simulink model "LinMotAct_total"  (R2019b)
settings: Solver=FixedStepAuto  StartTime=0.0  StopTime=inf  FixedStep=0.001  RelTol=1e-3  EnableMultiTasking=on
PostLoadFcn:
  | if any(exist('dsrtsu_mdlpostloadfcn', 'file') ~= 0), dsrtsu_mdlpostloadfcn('Execute', bdroot); end
values from neighbouring files (symbols this model uses):
  Ts_Outer = 0.1    [Working_model_LastVersion24_June.m]    (also in model_and_controller.m)
undefined symbols (not defined in the file or in its folder): denc_mi, denco13_dis_des, denF, numc_mi, numco13_dis_des, numF
libraries: rti3002t2lib x6, simulink x4, rtilibm x3, rti4201serlib x3
(part 1 of 2)
settings Model: DSRTSU_INTERNAL_RTI_VER=550  DSRTSU_INTERNAL_RTI_TYPE=rti1005  RTICANMMDATA=struct('GeneralSetupData',struct('modelroot','C:\Ball_and_Plate\Actuator_Control','generalsettings',struct('filesettings',struct('destfolder',struct('Name','RTICANMM_FILES','Check',1),'buildfolder',struct('Name','.','Check',1),'AbsDestfolder',struct('Name','C:\Ball_and_Plate\Actuator_Control\RTICANMM_FILES'),'AbsBuildfolder',struct('Name','C:\Ball_and_Plate\Actuator_Control'))),'options',struct('addpaths',1,'rmpaths',1,'addtrcexclusion',true,'cannavigator',struct('checkmonitoring',0),'show_usrtrc',0,'use_usrtrc',0),'advanced',struct('options',ones(1,100)),'MPSetup',{{}},'RTI',struct('Type','RTI1005','Ver','7.13','Date','02-Nov-2019'),'modelname','LinMotAct_total','block','LinMotAct_total'))  DSRTSU_INTERNAL_RTIFPGA=150  ExtModeArmWhenConnect=off  Creator=s060699  LastModifiedBy=20193994
settings SolverCC: AutoInsertRateTranBlk=on
settings DataIOCC: LimitDataPoints=on  SaveFormat=Array  SignalLoggingSaveFormat=ModelDataLogs  ReturnWorkspaceOutputs=off  SignalLoggingName=sigsOut
settings OptimizationCC: BlockReduction=off  ConditionallyExecuteInputs=off  OptimizeBlockIOStorage=off  BufferReuse=off  GlobalBufferReuse=off  ExpressionFolding=off  ExpressionDepthLimit=2147483647  LocalBlockOutputs=off  InitFltsAndDblsToZero=on  LifeSpan=inf  OptimizeDataStoreBuffers=off  BusAssignmentInplaceUpdate=off
settings DebuggingCC: SaveWithParameterizedLinksMsg=none  UnderspecifiedInitializationDetection=Classic  MergeDetectMultiDrivingBlocksExec=none  SignalResolutionControl=TryResolveAllWithWarning  MultiTaskDSMMsg=warning  MultiTaskCondExecSysMsg=none  FcnCallInpInsideContextMsg=warning  StateNameClashWarn=warning  SFUnexpectedBacktrackingDiag=warning  SFNoUnconditionalDefaultTransitionDiag=warning  SFExecutionAtInitializationDiag=none  ArithmeticOperatorsInVariantConditions=warning
settings HardwareCC: ProdBitPerPointer=32  ProdBitPerSizeT=32  ProdBitPerPtrDiffT=32  ProdLargestAtomicInteger=Integer  ProdEndianess=BigEndian  ProdWordSize=32  ProdHWDeviceType=Custom Processor->Custom  TargetIntDivRoundTo=Zero  TargetEndianess=BigEndian  TargetHWDeviceType=Custom Processor->Custom
settings ModelReferenceCC: PropagateSignalLabelsOutOfModel=off
settings SFSimCC: MATLABDynamicMemAlloc=off
settings RTWCC: Description=dSPACE DS1005 Hardware Platform  SystemTargetFile=rti1005.tlc  MakeCommand=make_rti  TemplateMakefile=rti1005.tmf  RTWVerbose=off  RetainRTWFile=on
settings CodeAppCC: CustomSymbolStrField=$H$N$M  CustomSymbolStrFcn=$R$H$N$M$F  StateflowObjectComments=on
settings STFCustomTargetCC: TargetFcnLib=ansi_tfl_tmw.mat  ParMdlRefBuildCompliant=on  CPPClassGenCompliant=on  SystemTargetFile=rti1005.tlc
settings GRTTargetCC: TargetFcnLib=ansi_tfl_tmw.mat  TargetLangStandard=C89/C90 (ANSI)  CompOptLevelCompliant=off  ConcurrentExecutionCompliant=off  CombineOutputUpdateFcns=off  MatFileLogging=off  UseToolchainInfoCompliant=off  ExtModeMexFile=rti_comm_2
settings ConfigComp: CovMetricSettings=dw  CovHtmlReporting=on  CovSaveCumulativeToWorkspaceVar=on  CovSaveSingleToWorkspaceVar=on

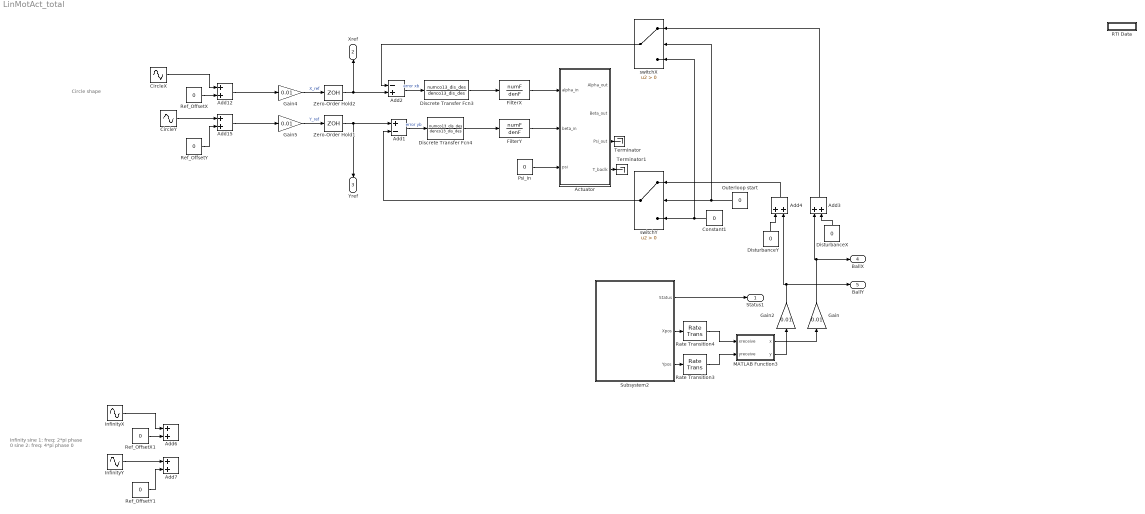
== system LinMotAct_total ==
  note: Infinity
      | sine 1: freq: 2*pi   phase 0
      | sine 2: freq: 4*pi   phase 0
  note: Circle shape
  Actuator : Subsystem
  Add1 : Sum  Inputs=+-
  Add{3..4,6..7,12,15} (6 alike) : Sum
  Add2 : Sum  Inputs=-+
  CircleX : Sin  Amplitude=0  Frequency=0.8  SampleTime=0
  CircleY : Sin  Amplitude=0  Frequency=0.8  Phase=pi/2  SampleTime=0
  Constant1 : Constant  Value=0
  Discrete Transfer Fcn3 : DiscreteTransferFcn  Numerator=numco13_dis_des  Denominator=denco13_dis_des
  Discrete Transfer Fcn4 : DiscreteTransferFcn  Numerator=numco13_dis_des  Denominator=denco13_dis_des
  DisturbanceX : Constant  Value=0
  DisturbanceY : Constant  Value=0
  FilterX : TransferFcn  Numerator=numF  Denominator=denF
  FilterY : TransferFcn  Numerator=numF  Denominator=denF
  Gain{,2,4..5} (4 alike) : Gain  Gain=0.01
  InfinityX : Sin  Amplitude=0  Frequency=1.41  SampleTime=0
  InfinityY : Sin  Amplitude=0  Frequency=2.82  SampleTime=0
  MATLAB Function3 : MATLAB Function  TreatAsAtomicUnit=on
  Outerloop start : Constant  Value=0
  Psi_in : Constant  Value=0
  RTI Data : Subsystem  Tag=struct('RTIDataServer',struct('RTIDataServerVs','2','RTIModelDescription','struct(''main'',''LinMotAct_total'',''sub'','''',''isMp'',0)'))  LoadFcn="if exist('rtidc'), try,  rtidc('DataHostBlockClbLoad', gcbh); catch, disp(['Warning: ''LoadFcn'' for RTI Data block failed: ' lasterr]); end, end,"  mask(RTI_DATA_HOST){}
      mask help:
      | RTI Data Block.
      | This block is used by RTI to store internal model-dependent data.
      | Please keep this block on the root level of the model. Deleting this block will result in data loss.
      |
      | NEVER DELETE OR COPY THIS BLOCK!
      settings: CopyFcn="if exist('rtidc'), try,  rtidc('DataHostBlockClbCopy', gcbh); catch, disp(['Warning: ''CopyFcn'' for RTI Data block failed: ' lasterr]); end, end,"  DeleteFcn="if exist('rtidc'), try,  rtidc('DataHostBlockClbDelete', gcbh); catch, disp(['Warning: ''DeleteFcn'' for RTI Data block failed: ' lasterr]); end, end,"  ModelCloseFcn="if exist('rtidc'), try,  rtidc('DataHostBlockClbModelClose', gcbh); catch, disp(['Warning: ''ModelCloseFcn'' for RTI Data block failed: ' lasterr]); end, end,"  PreSaveFcn="if exist('rtidc'), try,  rtidc('DataHostBlockClbPreSave', gcbh); catch, disp(['Warning: ''PreSaveFcn'' for RTI Data block failed: ' lasterr]); end, end,"  PostSaveFcn="if exist('rtidc'), try,  rtidc('DataHostBlockClbPostSave', gcbh); catch, disp(['Warning: ''PostSaveFcn'' for RTI Data block failed: ' lasterr]); end, end,"  NameChangeFcn="if exist('rtidc'), try,  rtidc('DataHostBlockClbNameChange', gcbh); catch, disp(['Warning: ''NameChangeFcn'' for RTI Data block failed: ' lasterr]); end, end,"
      mask Help:
      | RTI Data Block.
      | This block is used by RTI to store internal model-dependent data.
      | Please keep this block on the root level of the model. Deleting this block will result in data loss.
      | 
      | NEVER DELETE OR COPY THIS BLOCK!
      mask Display:
      | text(0.5, 0.5, 'RTI Data', 'HorizontalAlignment', 'center');
      | plot([1 0]);
  Rate Transition3 : RateTransition  Deterministic=off  OutPortSampleTimeMultiple=Ts_Outer  OutPortSampleTime=Ts_Outer
  Rate Transition4 : RateTransition  Deterministic=off  OutPortSampleTimeMultiple=Ts_Outer  OutPortSampleTime=Ts_Outer
  Ref_OffsetX : Constant  Value=0
  Ref_OffsetX1 : Constant  Value=0
  Ref_OffsetY : Constant  Value=0
  Ref_OffsetY1 : Constant  Value=0
  Subsystem2 : Subsystem
  Terminator : Terminator
  Terminator1 : Terminator
  Zero-Order Hold1 : ZeroOrderHold  SampleTime=Ts_Outer
  Zero-Order Hold2 : ZeroOrderHold  SampleTime=Ts_Outer
  switchX : Switch  Criteria=u2 > Threshold
  switchY : Switch  Criteria=u2 > Threshold
  Status1 : Outport
  Xref : Outport  Port=2
  Yref : Outport  Port=3
  BallX : Outport  Port=4
  BallY : Outport  Port=5
  wires:
  Ref_OffsetY/1 -> Add15/2
  CircleY/1 -> Add15/1
  Ref_OffsetX/1 -> Add12/2
  CircleX/1 -> Add12/1
  Gain4/1 -> Zero-Order Hold2/1  "X_ref"
  Gain5/1 -> Zero-Order Hold1/1  "Y_ref"
  Psi_in/1 -> Actuator/3(psi)
  Actuator/3(Psi_out) -> Terminator/1
  Actuator/4(T_baclk) -> Terminator1/1
  Subsystem2/1(Status) -> Status1/1
  Subsystem2/3(Ypos) -> Rate Transition3/1
  Subsystem2/2(Xpos) -> Rate Transition4/1
  Rate Transition3/1 -> MATLAB Function3/2(yreceive)
  Rate Transition4/1 -> MATLAB Function3/1(xreceive)
  MATLAB Function3/1(x) -> Gain/1
  Add2/1 -> Discrete Transfer Fcn3/1  "error xb"
  Add1/1 -> Discrete Transfer Fcn4/1  "error yb"
  Zero-Order Hold2/1 -> Add2/2, Xref/1
  Zero-Order Hold1/1 -> Add1/1, Yref/1
  Outerloop start/1 -> switchY/2, switchX/2
  Constant1/1 -> switchX/3, switchY/3
  Gain/1 -> Add3/1, BallX/1
  MATLAB Function3/2(y) -> Gain2/1
  DisturbanceX/1 -> Add3/2
  DisturbanceY/1 -> Add4/1
  switchY/1 -> Add1/2
  switchX/1 -> Add2/1
  Add4/1 -> switchY/1
  Add3/1 -> switchX/1
  Gain2/1 -> Add4/2, BallY/1
  FilterX/1 -> Actuator/1(alpha_in)
  FilterY/1 -> Actuator/2(beta_in)
  Ref_OffsetX1/1 -> Add6/2
  InfinityX/1 -> Add6/1
  Ref_OffsetY1/1 -> Add7/2
  InfinityY/1 -> Add7/1
  Add12/1 -> Gain4/1
  Add15/1 -> Gain5/1
  Discrete Transfer Fcn3/1 -> FilterX/1
  Discrete Transfer Fcn4/1 -> FilterY/1

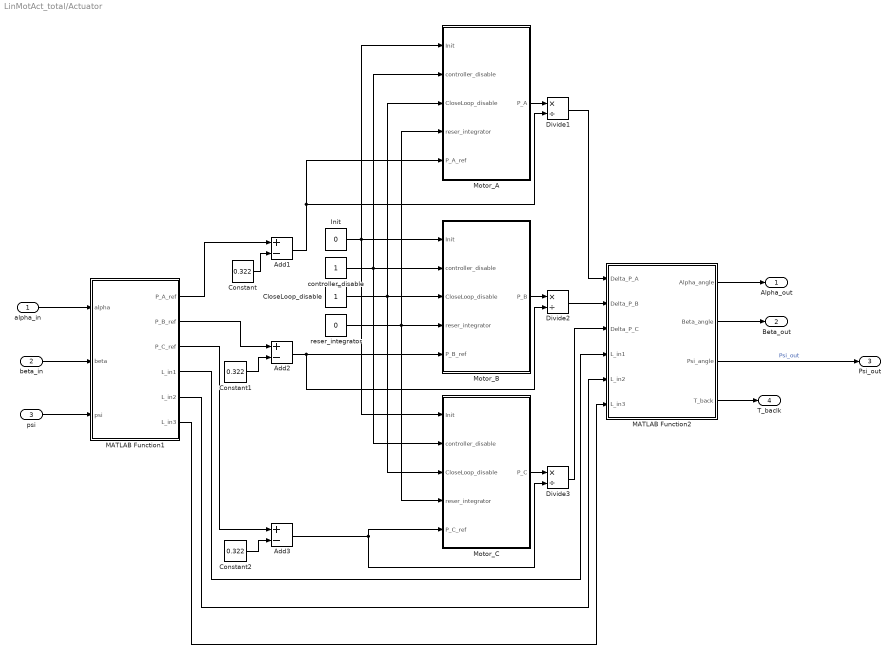
== system LinMotAct_total/Actuator ==
  alpha_in : Inport
  beta_in : Inport  Port=2
  psi : Inport  Port=3
  Add1 : Sum  Inputs=+-
  Add2 : Sum  Inputs=+-
  Add3 : Sum  Inputs=+-
  CloseLoop_disable : Constant
  Constant : Constant  Value=0.322
  Constant1 : Constant  Value=0.322
  Constant2 : Constant  Value=0.322
  Divide1 : Product  Inputs=*/
  Divide2 : Product  Inputs=*/
  Divide3 : Product  Inputs=*/
  "Init " : Constant  Value=0
  MATLAB Function1 : MATLAB Function  TreatAsAtomicUnit=on
  MATLAB Function2 : MATLAB Function  TreatAsAtomicUnit=on
  Motor_A : Subsystem
  Motor_B : Subsystem
  Motor_C : Subsystem
  controller_disable : Constant
  reser_integrator : Constant  Value=0
  Alpha_out : Outport
  Beta_out : Outport  Port=2
  Psi_out : Outport  Port=3
  T_baclk : Outport  Port=4
  wires:
  Motor_B/1(P_B) -> Divide2/1
  "Init "/1 -> Motor_C/1(Init), Motor_A/1(Init), Motor_B/1(Init)
  Divide3/1 -> MATLAB Function2/3(Delta_P_C)
  controller_disable/1 -> Motor_A/2(controller_disable), Motor_B/2(controller_disable), Motor_C/2(controller_disable)
  Add3/1 -> Motor_C/5(P_C_ref), Divide3/2
  MATLAB Function1/1(P_A_ref) -> Add1/1
  reser_integrator/1 -> Motor_A/4(reser_integrator), Motor_C/4(reser_integrator), Motor_B/4(reser_integrator)
  MATLAB Function1/3(P_C_ref) -> Add3/1
  MATLAB Function1/5(L_in2) -> MATLAB Function2/5(L_in2)
  Divide1/1 -> MATLAB Function2/1(Delta_P_A)
  Motor_C/1(P_C) -> Divide3/1
  MATLAB Function2/1(Alpha_angle) -> Alpha_out/1
  psi/1 -> MATLAB Function1/3(psi)
  Add2/1 -> Divide2/2, Motor_B/5(P_B_ref)
  Motor_A/1(P_A) -> Divide1/1
  MATLAB Function2/4(T_back) -> T_baclk/1
  Add1/1 -> Motor_A/5(P_A_ref), Divide1/2
  Constant1/1 -> Add2/2
  beta_in/1 -> MATLAB Function1/2(beta)
  Constant/1 -> Add1/2
  Constant2/1 -> Add3/2
  Divide2/1 -> MATLAB Function2/2(Delta_P_B)
  MATLAB Function1/6(L_in3) -> MATLAB Function2/6(L_in3)
  CloseLoop_disable/1 -> Motor_A/3(CloseLoop_disable), Motor_C/3(CloseLoop_disable), Motor_B/3(CloseLoop_disable)
  MATLAB Function1/2(P_B_ref) -> Add2/1
  MATLAB Function1/4(L_in1) -> MATLAB Function2/4(L_in1)
  MATLAB Function2/2(Beta_angle) -> Beta_out/1
  MATLAB Function2/3(Psi_angle) -> Psi_out/1  "Psi_out"
  alpha_in/1 -> MATLAB Function1/1(alpha)

== system LinMotAct_total/RTI Data ==
  RTI Data Store : Subsystem  Tag="struct('private',struct('version',struct('dsVer',uint32(2),'dsVerCreation',uint32(2),'RTI',struct('ver','7.13','type','RTI1005')),'access',struct('type','Model','isPerm',1,'created',['07-Jul-2020 15:56:35'],'modified',['31-Jul-2020 14:12:37'],'location','')),'public',struct('main',struct('data',[]),'sub',struct('name',{{'LinMotAct_total'}},'data',{{struct('TH',struct('thTaskInfo',struct('taskType',{'TIMER','HWINT','TMRINT','SWINT','GLINT'},'tasksNumOf',{2,0,0,0,0},'srcIds',{{'TIMERA','TIMERA2'},{},{},{},{}},'taskNames',{{['Timer Task 1'],['Timer Task 2']},{},{},{},{}})),'th_tc',struct('dataType',{'TASK','TASK'},'taskGroupId',{'',''},'taskGroupList',{{},{}},'taskSchedulingPolicy',{'FCFS','FCFS'},'taskType',{'TIMER','TIMER'},'blkh',{-1,-1},'srcId',{'TIMERA','TIMERA2'},'srcSgnName',{['Timer A interrupt'],['Timer Task 1']},'srcCpuName',{'',''},'taskName',{['Timer Task 1  [0.001] s'],['Timer Task 2  [0.1] s']},'taskNameDisplayExt',{'',''},'smplTime',{0.001,0.1},'smplTimeOffs',{0,0},'hasFixedPriority',{0,0},'priority',{1,2},'hasFixedOvc',{0,0},'ovcType',{1,1},'ovcMax',{1,1}),'tc_th',struct('dataType',{'TASK','TASK'},'taskGroupId',{'',''},'taskGroupList',{{},{}},'taskSchedulingPolicy',{'FCFS','FCFS'},'taskType',{'TIMER','TIMER'},'blkh',{-1,-1},'srcId',{'TIMERA','TIMERA2'},'srcSgnName',{['Timer A interrupt'],['Timer Task 1']},'srcCpuName',{'',''},'taskName',{['Timer Task 1  [0.001] s'],['Timer Task 2  [0.1] s']},'taskNameDisplayExt',{'',''},'smplTime',{0.001,0.1},'smplTimeOffs',{0,0},'hasFixedPriority',{0,0},'priority',{1,2},'hasFixedOvc',{0,0},'ovcType',{1,1},'ovcMax',{1,1}))}})))"  mask(RTI_DATA_STORE){}
      mask help:
      | RTI Data Store Block. This block is used by RTI to store internal model dependent data. Deleting this block will result in data loss.
      |
      | NEVER DELETE, COPY, OR MODIFY THIS BLOCK!
      mask Help:
      | RTI Data Store Block. This block is used by RTI to store internal model dependent data. Deleting this block will result in data loss.
      | 
      | NEVER DELETE, COPY, OR MODIFY THIS BLOCK!
      mask Display: text(0.5, 0.5, ' ', 'HorizontalAlignment', 'center');

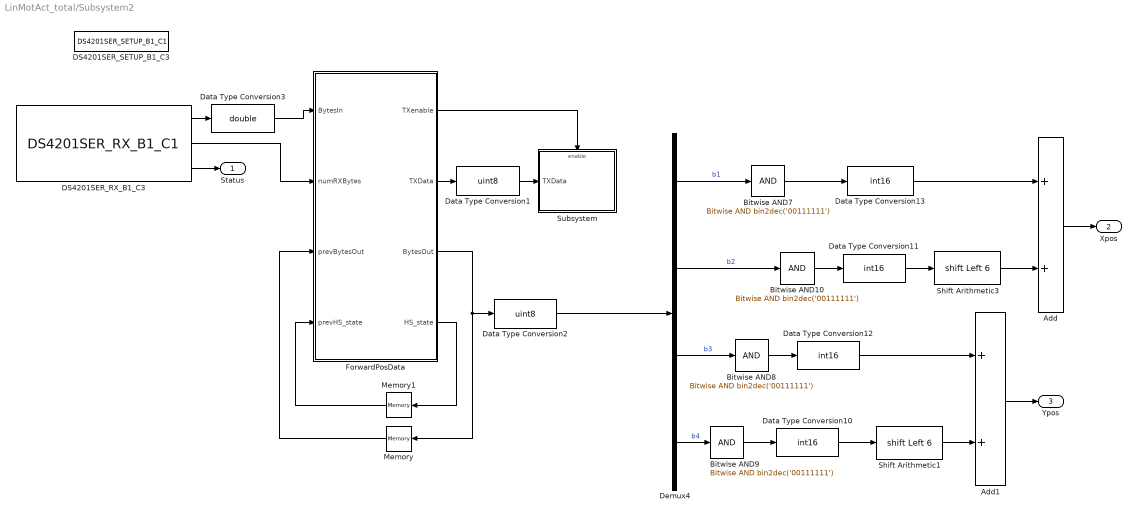
== system LinMotAct_total/Subsystem2 ==
  Add : Sum
  Add1 : Sum
  Bitwise AND{7..10} (4 alike) : simulink/Logic and Bit Operations/Bitwise Operator  logicop=AND  UseBitMask=on  BitMask=bin2dec('00111111')  BitMaskRealWorld=Stored Integer
  DS4201SER_RX_B1_C3 : rti4201serlib/DS4201SER_RX_B1_C1  Reserved1=[]  Reserved2=[]  Reserved3=[]  Reserved4=[]  DSProperties=struct('RTI',struct('IOBoardType',{{'DS4201','SER'}},'SlaveProcessor','NONE','Version',uint32(1),'BlockType',struct('isSLSource',uint8(1),'isSLSink',uint8(1),'isHWSource',uint8(0),'isHWSink',uint8(1),'isSetup',uint8(0),'isInline',uint8(1),'isNonInline',uint8(0),'isInterrupt',uint8(0),'isChannelwise',uint8(1)),'UnitType','GENSER','Identifier','RECEIVE','DialogType','ML','BlockSet','NONE'))  RTIBlockInterface=struct('BlockName',struct('Token',{{'DS4201SER_RX_B','_C'}},'BlockParam',{{'BoardNo','ChannelNo'}}),'InputPortsWidth',int32(1),'InputPortsActive',0,'InputPortsDataType',{{'SS_UINT32'}},'InputPortsName',{{'NumBytes'}},'OutputPortsWidth',int32([4 1 1]),'OutputPortsActive',[1 1 1],'OutputPortsDataType',{{'SS_UINT8','SS_UINT32','SS_INT32'}},'OutputPortsName',{{'RXBytes','NumRXBytes','Status'}},'BlockDisplay',{{['Serial Receive'],'center'}},'IconTransparency','on','ParameterTunableNames',{{'BytesRefNumOf'}},'InitLevel',2,'DialogFcn','guigenserreceive','MaskDescription',['To read data from the UART SW FIFO.'])  RTIBlockParameters=struct('BoardNo',{{1,'ON',[1 16]}},'ChannelNo',{{3,'ON',[1 4]}},'ChannelNumOf',{{4,'OFF',[]}},'ReceptionDataMode',{{2,'OFF',[]}},'ParamTunableMode',{{1,'OFF',[]}},'BytesRefNumOfT',{{'4','OFF',[1 inf]}},'BytesRefNumOfNT',{{'4','OFF',[1 inf]}},'BytesRefNumOfMax',{{'4','OFF',[1 inf]}},'BytesRefNumOfMode',{{1,'OFF',[]}},'BytesActNumOfMode',{{1,'OFF',[]}},'ReceptionStatusMode',{{1,'OFF',[]}},'FifoSizeDefault',{{64,'OFF',[]}},'TLCFileName',{{'rtigenserreceive','OFF',[]}})  RTISFcnParameters=struct('BoardNo','double','ChannelNo','double','ChannelNumOf','double','ReceptionDataMode','double','ParamTunableMode','double','BytesRefNumOfT','double','BytesRefNumOfNT','double','BytesRefNumOfMax','double','BytesRefNumOfMode','double','BytesActNumOfMode','double','ReceptionStatusMode','double','TLCFileName','char')  RTIBlockParaDefault=struct('BoardNo',1,'ChannelNo',1,'ChannelNumOf',4,'ReceptionDataMode',1,'ParamTunableMode',1,'BytesRefNumOfT',1,'BytesRefNumOfNT',1,'BytesRefNumOfMax',1,'BytesRefNumOfMode',0,'BytesActNumOfMode',1,'ReceptionStatusMode',1,'FifoSizeDefault',64,'TLCFileName','rtigenserreceive')
  DS4201SER_SETUP_B1_C3 : rti4201serlib/DS4201SER_SETUP_B1_C1  Reserved1=[]  Reserved2=[]  Reserved3=[]  Reserved4=[]  DSProperties=struct('RTI',struct('Version',uint32(2),'IOBoardType',{{'DS4201','SER'}},'SlaveProcessor','NONE','BlockType',struct('isSLSource',uint8(0),'isSLSink',uint8(0),'isHWSource',uint8(0),'isHWSink',uint8(0),'isSetup',uint8(1),'isInline',uint8(1),'isNonInline',uint8(0),'isInterrupt',uint8(0),'isChannelwise',uint8(1)),'UnitType','GENSER','Identifier','SETUP','DialogType','ML','BlockSet','NONE'))  RTIBlockInterface=struct('BlockName',struct('Token',{{'DS4201SER_SETUP_B','_C'}},'BlockParam',{{'BoardNo','ChannelNo'}}),'BlockDisplay',{{['Serial Setup'],'center'}},'IconTransparency','off','ParameterTunableNames',{{}},'InitLevel',1,'DialogFcn','guigensersetup','MaskDescription',['To set the global specifications for the UART interface.'])  RTIBlockParameters=struct('ParityMode',{{1,'OFF',[1 3]}},'TransceiverMode',{{[3;1;3;1],'OFF',[]}},'QuartzFrequency',{{'24000000','OFF',[]}},'BoardNo',{{1,'ON',[1 16]}},'ChannelNo',{{3,'ON',[1 4]}},'ChannelNumOf',{{4,'OFF',[]}},'BaudRate',{{'9600','OFF',[]}},'DataBitsNumOf',{{4,'OFF',[1 4]}},'StopBitsNumOf',{{1,'OFF',[1 3]}},'ReceiveIntLevelUart',{{2,'OFF',[1 4]}},'AutoflowMode',{{0,'OFF',[]}},'FifoSize',{{'64','OFF',[]}},'ReceiveIntLevelFifo',{{0,'OFF',[]}},'FifoOverrunMode',{{2,'OFF',[]}},'FifoBlockSize',{{'4','OFF',[]}},'TermMode',{{0,'OFF',[]}},'TLCFileName',{{'rtigensersetup','OFF',[]}})  RTISFcnParameters=struct('BoardNo','double','ChannelNo','double','ChannelNumOf','double','BaudRate','double','DataBitsNumOf','double','StopBitsNumOf','double','ParityMode','double','TransceiverMode','double','ReceiveIntLevelUart','double','AutoflowMode','double','FifoSize','double','ReceiveIntLevelFifo','double','FifoBlockSize','double','TermMode','double','QuartzFrequency','double','TLCFileName','char')  RTIBlockParaDefault=struct('ParityMode',1,'TransceiverMode',[1;1;1;1],'QuartzFrequency',1843200,'BoardNo',1,'ChannelNo',1,'ChannelNumOf',4,'BaudRate',115200,'DataBitsNumOf',4,'StopBitsNumOf',1,'ReceiveIntLevelUart',4,'AutoflowMode',0,'FifoSize',64,'ReceiveIntLevelFifo',0,'FifoOverrunMode',1,'FifoBlockSize',0,'TermMode',1,'TLCFileName','rtigensersetup')
  Data Type Conversion1 : DataTypeConversion  OutDataTypeStr=uint8
  Data Type Conversion{10..13} (4 alike) : DataTypeConversion  OutDataTypeStr=int16
  Data Type Conversion2 : DataTypeConversion  OutDataTypeStr=uint8
  Data Type Conversion3 : DataTypeConversion  OutDataTypeStr=double
  Demux4 : Demux
  ForwardPosData : MATLAB Function  TreatAsAtomicUnit=on
  Memory : Memory  InitialCondition=[0 0 0 0]
  Memory1 : Memory
  Shift Arithmetic1 : ArithShift  BitShiftNumber=6  BitShiftDirection=Left
  Shift Arithmetic3 : ArithShift  BitShiftNumber=6  BitShiftDirection=Left
  Subsystem : Subsystem
  Status : Outport
  Xpos : Outport  Port=2
  Ypos : Outport  Port=3
  wires:
  Bitwise AND8/1 -> Data Type Conversion12/1
  Bitwise AND7/1 -> Data Type Conversion13/1
  Add/1 -> Xpos/1
  Add1/1 -> Ypos/1
  Bitwise AND10/1 -> Data Type Conversion11/1
  Bitwise AND9/1 -> Data Type Conversion10/1
  Data Type Conversion11/1 -> Shift Arithmetic3/1
  Data Type Conversion10/1 -> Shift Arithmetic1/1
  Data Type Conversion13/1 -> Add/1
  Data Type Conversion12/1 -> Add1/1
  Shift Arithmetic3/1 -> Add/2
  Shift Arithmetic1/1 -> Add1/2
  DS4201SER_RX_B1_C3/2 -> ForwardPosData/2(numRXBytes)
  DS4201SER_RX_B1_C3/3 -> Status/1
  ForwardPosData/3(BytesOut) -> Data Type Conversion2/1, Memory/1
  Memory/1 -> ForwardPosData/3(prevBytesOut)
  DS4201SER_RX_B1_C3/1 -> Data Type Conversion3/1
  ForwardPosData/4(HS_state) -> Memory1/1
  Memory1/1 -> ForwardPosData/4(prevHS_state)
  ForwardPosData/2(TXData) -> Data Type Conversion1/1
  ForwardPosData/1(TXenable) -> Subsystem/Enable
  Demux4/1 -> Bitwise AND7/1  "b1"
  Demux4/2 -> Bitwise AND10/1  "b2"
  Demux4/3 -> Bitwise AND8/1  "b3"
  Demux4/4 -> Bitwise AND9/1  "b4"
  Data Type Conversion1/1 -> Subsystem/1(TXData)
  Data Type Conversion2/1 -> Demux4/1
  Data Type Conversion3/1 -> ForwardPosData/1(BytesIn)

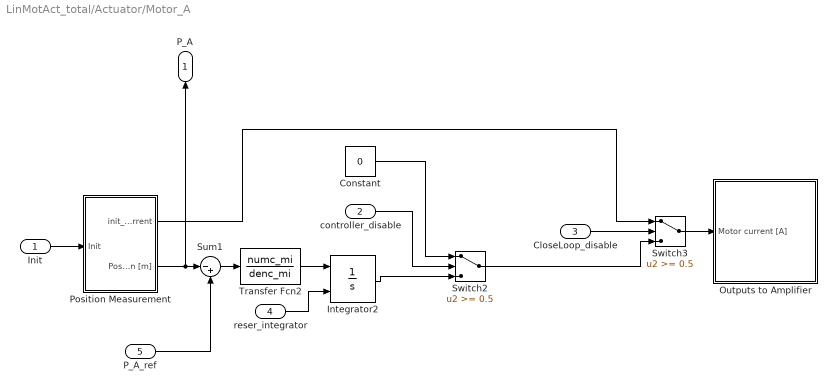
== system LinMotAct_total/Actuator/Motor_A ==
  Init : Inport
  controller_disable : Inport  Port=2
  CloseLoop_disable : Inport  Port=3
  reser_integrator : Inport  Port=4
  P_A_ref : Inport  Port=5
  Constant : Constant  Value=0
  Integrator2 : Integrator  ExternalReset=rising  LimitOutput=on  UpperSaturationLimit=2.7  LowerSaturationLimit=-2.7
  Outputs to Amplifier : Subsystem  TreatAsAtomicUnit=on
  Position Measurement : Subsystem  TreatAsAtomicUnit=on
  Sum1 : Sum  Inputs=|-+  SaturateOnIntegerOverflow=on
  Switch2 : Switch  Threshold=0.5
  Switch3 : Switch  Threshold=0.5
  Transfer Fcn2 : TransferFcn  Numerator=numc_mi  Denominator=denc_mi
  P_A : Outport
  wires:
  Integrator2/1 -> Switch2/3
  Switch3/1 -> Outputs to Amplifier/1(Motor current [A])
  Position Measurement/2(Position [m]) -> P_A/1, Sum1/1
  Position Measurement/1(init_current) -> Switch3/1
  Switch2/1 -> Switch3/3
  CloseLoop_disable/1 -> Switch3/2
  reser_integrator/1 -> Integrator2/2
  Sum1/1 -> Transfer Fcn2/1
  Constant/1 -> Switch2/1
  Transfer Fcn2/1 -> Integrator2/1
  controller_disable/1 -> Switch2/2
  P_A_ref/1 -> Sum1/2
  Init/1 -> Position Measurement/1(Init)

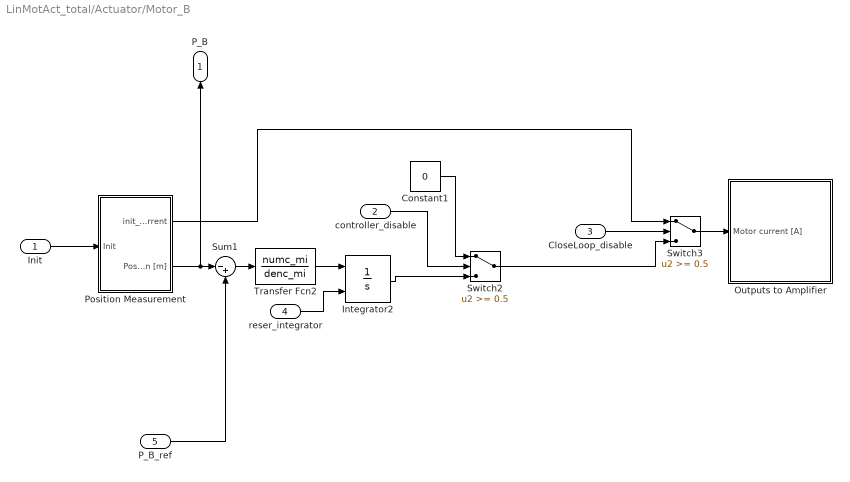
== system LinMotAct_total/Actuator/Motor_B ==
  Init : Inport
  controller_disable : Inport  Port=2
  CloseLoop_disable : Inport  Port=3
  reser_integrator : Inport  Port=4
  P_B_ref : Inport  Port=5
  Constant1 : Constant  Value=0
  Integrator2 : Integrator  ExternalReset=rising  LimitOutput=on  UpperSaturationLimit=2.7  LowerSaturationLimit=-2.7
  Outputs to Amplifier : Subsystem  TreatAsAtomicUnit=on
  Position Measurement : Subsystem  TreatAsAtomicUnit=on
  Sum1 : Sum  Inputs=|-+  SaturateOnIntegerOverflow=on
  Switch2 : Switch  Threshold=0.5
  Switch3 : Switch  Threshold=0.5
  Transfer Fcn2 : TransferFcn  Numerator=numc_mi  Denominator=denc_mi
  P_B : Outport
  wires:
  Integrator2/1 -> Switch2/3
  Switch3/1 -> Outputs to Amplifier/1(Motor current [A])
  Position Measurement/2(Position [m]) -> P_B/1, Sum1/1
  Position Measurement/1(init_current) -> Switch3/1
  Switch2/1 -> Switch3/3
  CloseLoop_disable/1 -> Switch3/2
  reser_integrator/1 -> Integrator2/2
  Sum1/1 -> Transfer Fcn2/1
  Transfer Fcn2/1 -> Integrator2/1
  controller_disable/1 -> Switch2/2
  P_B_ref/1 -> Sum1/2
  Constant1/1 -> Switch2/1
  Init/1 -> Position Measurement/1(Init)

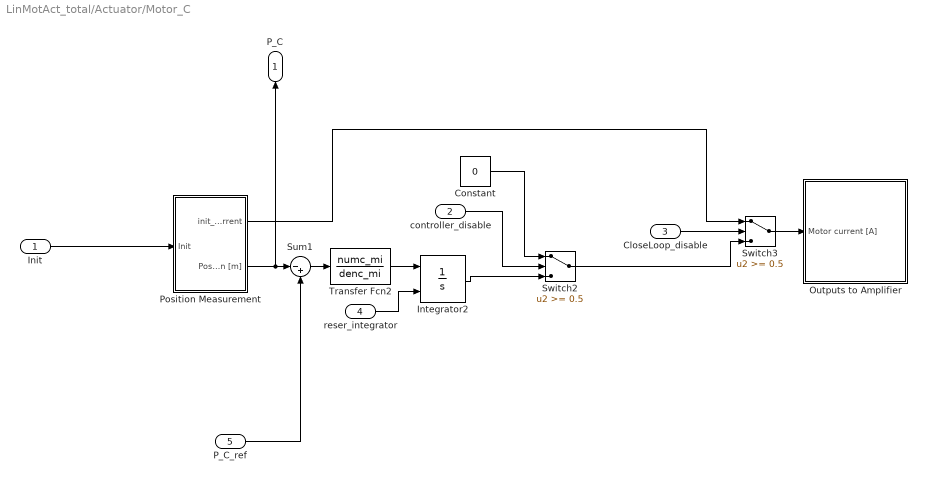
== system LinMotAct_total/Actuator/Motor_C ==
  Init : Inport
  controller_disable : Inport  Port=2
  CloseLoop_disable : Inport  Port=3
  reser_integrator : Inport  Port=4
  P_C_ref : Inport  Port=5
  Constant : Constant  Value=0
  Integrator2 : Integrator  ExternalReset=rising  LimitOutput=on  UpperSaturationLimit=2.7  LowerSaturationLimit=-2.7
  Outputs to Amplifier : Subsystem  TreatAsAtomicUnit=on
  Position Measurement : Subsystem  TreatAsAtomicUnit=on
  Sum1 : Sum  Inputs=|-+  SaturateOnIntegerOverflow=on
  Switch2 : Switch  Threshold=0.5
  Switch3 : Switch  Threshold=0.5
  Transfer Fcn2 : TransferFcn  Numerator=numc_mi  Denominator=denc_mi
  P_C : Outport
  wires:
  Integrator2/1 -> Switch2/3
  Switch3/1 -> Outputs to Amplifier/1(Motor current [A])
  Position Measurement/2(Position [m]) -> P_C/1, Sum1/1
  Position Measurement/1(init_current) -> Switch3/1
  Switch2/1 -> Switch3/3
  CloseLoop_disable/1 -> Switch3/2
  reser_integrator/1 -> Integrator2/2
  Sum1/1 -> Transfer Fcn2/1
  Constant/1 -> Switch2/1
  Transfer Fcn2/1 -> Integrator2/1
  controller_disable/1 -> Switch2/2
  P_C_ref/1 -> Sum1/2
  Init/1 -> Position Measurement/1(Init)

== system LinMotAct_total/RTI Data/RTI Data Store ==
  RTI Data Store : Subsystem  mask(RTI_DATA_STORE){}
      mask help:
      | RTI Data Store Block. This block is used by RTI to store internal model dependent data. Deleting this block will result in data loss.
      |
      | NEVER DELETE, COPY, OR MODIFY THIS BLOCK!
      mask Help:
      | RTI Data Store Block. This block is used by RTI to store internal model dependent data. Deleting this block will result in data loss.
      | 
      | NEVER DELETE, COPY, OR MODIFY THIS BLOCK!
      mask Display: text(0.5, 0.5, ' ', 'HorizontalAlignment', 'center');

== system LinMotAct_total/Subsystem2/Subsystem ==
  TXData : Inport
  Enable : EnablePort
  DS4201SER_TX_B1_C3 : rti4201serlib/DS4201SER_TX_B1_C1  Reserved1=[]  Reserved2=[]  Reserved3=[]  Reserved4=[]  DSProperties=struct('RTI',struct('IOBoardType',{{'DS4201','SER'}},'SlaveProcessor','NONE','Version',uint32(1),'BlockType',struct('isSLSource',uint8(1),'isSLSink',uint8(1),'isHWSource',uint8(1),'isHWSink',uint8(0),'isSetup',uint8(0),'isInline',uint8(1),'isNonInline',uint8(0),'isInterrupt',uint8(0),'isChannelwise',uint8(1)),'UnitType','GENSER','Identifier','TRANSMIT','DialogType','ML','BlockSet','NONE'))  RTIBlockInterface=struct('BlockName',struct('Token',{{'DS4201SER_TX_B','_C'}},'BlockParam',{{'BoardNo','ChannelNo'}}),'InputPortsWidth',int32([1 1]),'InputPortsActive',[1 0],'InputPortsDataType',{{'SS_UINT8','SS_UINT32'}},'InputPortsName',{{'TXBytes','NumBytes'}},'OutputPortsWidth',int32([1 1]),'OutputPortsActive',[1 1],'OutputPortsDataType',{{'SS_UINT32','SS_INT32'}},'OutputPortsName',{{'NumTXBytes','Status'}},'BlockDisplay',{{['Serial Transmit'],'center'}},'IconTransparency','on','ParameterTunableNames',{{'BytesRefNumOf'}},'InitLevel',2,'DialogFcn','guigensertransmit','MaskDescription',['To write data to the UART SW FIFO.'])  RTIBlockParameters=struct('BoardNo',{{1,'ON',[1 16]}},'ChannelNo',{{3,'ON',[1 4]}},'ChannelNumOf',{{4,'OFF',[]}},'TransmitFifoOverrunMode',{{1,'OFF',[]}},'ParamTunableMode',{{1,'OFF',[]}},'BytesRefNumOfT',{{'1','OFF',[1 inf]}},'BytesRefNumOfNT',{{'1','OFF',[1 inf]}},'BytesRefNumOfMax',{{'1','OFF',[1 inf]}},'BytesRefNumOfMode',{{1,'OFF',[]}},'BytesActNumOfMode',{{1,'OFF',[]}},'TransmissionStatusMode',{{1,'OFF',[]}},'FifoSizeDefault',{{64,'OFF',[]}},'TLCFileName',{{'rtigensertransmit','OFF',[]}})  RTISFcnParameters=struct('BoardNo','double','ChannelNo','double','ChannelNumOf','double','TransmitFifoOverrunMode','double','ParamTunableMode','double','BytesRefNumOfT','double','BytesRefNumOfNT','double','BytesRefNumOfMax','double','BytesRefNumOfMode','double','BytesActNumOfMode','double','TransmissionStatusMode','double','TLCFileName','char')  RTIBlockParaDefault=struct('BoardNo',1,'ChannelNo',1,'ChannelNumOf',4,'TransmitFifoOverrunMode',1,'ParamTunableMode',1,'BytesRefNumOfT',1,'BytesRefNumOfNT',1,'BytesRefNumOfMax',1,'BytesRefNumOfMode',0,'BytesActNumOfMode',1,'TransmissionStatusMode',1,'FifoSizeDefault',64,'TLCFileName','rtigensertransmit')
  Terminator : Terminator
  Terminator1 : Terminator
  wires:
  DS4201SER_TX_B1_C3/2 -> Terminator1/1
  DS4201SER_TX_B1_C3/1 -> Terminator/1
  TXData/1 -> DS4201SER_TX_B1_C3/1

== system LinMotAct_total/Actuator/Motor_A/Outputs to Amplifier ==
  Motor current [A] : Inport
  Current2V : Gain  Gain=10/3  SaturateOnIntegerOverflow=on  OutDataTypeStr=Inherit: Same as input  ParamDataTypeStr=Inherit: Same as input
  DS2102_B1 : rtilibm/DS2102/DS2102_B1  BoardNo=1  Range=[10 10 10 10 10 10]  IOErrorMode=[1 1 1 1 1 1]  DeglitcherMode=[0 0 0 0 0 0]  InitValue=[0 0 0 0 0 0]  TermMode=[1 1 1 1 1 1]  TermValue=[0 0 0 0 0 0]  DialogFcn=gui2102  UnitName={'DS2102_B'}  UnitValues={ 1 }  DSProperties=struct('RTI',struct('Version',uint32(1),'BlockType',struct('isSLSource',uint8(0),'isSLSink',uint8(1),'isHWSource',uint8(0),'isHWSink',uint8(1),'isSetup',uint8(0),'isInline',uint8(1),'isNonInline',uint8(0),'isInterrupt',uint8(0),'isChannelwise',uint8(0)),'IOBoardType','DS2102','UnitType','DAC','Identifier','DAC','DialogType','ML','BlockSet','NONE','SlaveProcessor','NONE'))
      settings: SourceProductName=dSPACE RTI1005
  DSPscale : Gain  Gain=1/10  SaturateOnIntegerOverflow=on  OutDataTypeStr=Inherit: Same as input  ParamDataTypeStr=Inherit: Same as input
  Saturation : Saturate  UpperLimit=3  LowerLimit=-3
  wires:
  Saturation/1 -> Current2V/1
  Current2V/1 -> DSPscale/1
  Motor current [A]/1 -> Saturation/1
  DSPscale/1 -> DS2102_B1/1

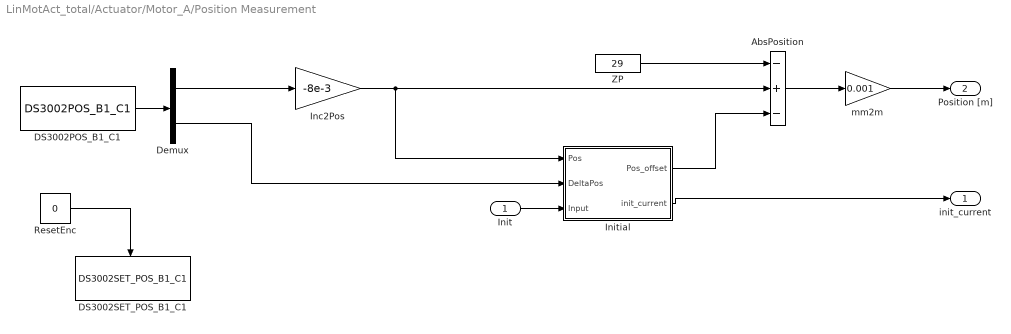
== system LinMotAct_total/Actuator/Motor_A/Position Measurement ==
  Init : Inport
  AbsPosition : Sum  Inputs=-+-  SaturateOnIntegerOverflow=on
  "DS3002POS_B1_C1 " : rti3002t2lib/DS3002POS_B1_C1  BoardNo=1  ChannelNo=1  LineSubdivNumOf=1  Reserved1=[]  Reserved2=[]  Reserved3=[]  Reserved4=[]  DialogFcn=gui3002pos_c_t2  UnitName={'DS3002POS_B', '_C'}  UnitValues="{ 1  1 }"  DSProperties=struct('RTI',struct('Version',uint32(1),'BlockType',struct('isSLSource',uint8(1),'isSLSink',uint8(0),'isHWSource',uint8(1),'isHWSink',uint8(0),'isSetup',uint8(0),'isInline',uint8(1),'isNonInline',uint8(0),'isInterrupt',uint8(0),'isChannelwise',uint8(1)),'IOBoardType','DS3002','UnitType','ENC','Identifier','ENCPOSCHT2','DialogType','ML','BlockSet','NONE','SlaveProcessor','NONE'))
  "DS3002SET_POS_B1_C1 " : rti3002t2lib/DS3002SET_POS_B1_C1  BoardNo=1  ChannelNo=1  PositionSetValue=0  Reserved1=[]  Reserved2=[]  Reserved3=[]  Reserved4=[]  DialogFcn=gui3002set_pos_c_t2  UnitName={'DS3002SET_POS_B', '_C'}  UnitValues="{ 1  1 }"  DSProperties=struct('RTI',struct('Version',uint32(1),'BlockType',struct('isSLSource',uint8(0),'isSLSink',uint8(1),'isHWSource',uint8(0),'isHWSink',uint8(0),'isSetup',uint8(0),'isInline',uint8(1),'isNonInline',uint8(0),'isInterrupt',uint8(0),'isChannelwise',uint8(1)),'IOBoardType','DS3002','UnitType','ENC','Identifier','ENCSETPOST2','DialogType','ML','BlockSet','NONE','SlaveProcessor','NONE'))
  Demux : Demux  Outputs=2
  Inc2Pos : Gain  Gain=-8e-3  SaturateOnIntegerOverflow=on  OutDataTypeStr=Inherit: Same as input  ParamDataTypeStr=Inherit: Same as input
  Initial : Subsystem
  ResetEnc : Constant  Value=0
  ZP : Constant  Value=29
  mm2m : Gain  Gain=0.001
  init_current : Outport  VectorParamsAs1DForOutWhenUnconnected=off
  Position [m] : Outport  Port=2  VectorParamsAs1DForOutWhenUnconnected=off
  wires:
  Demux/1 -> Inc2Pos/1
  AbsPosition/1 -> mm2m/1
  Inc2Pos/1 -> Initial/1(Pos), AbsPosition/2
  Initial/2(init_current) -> init_current/1
  mm2m/1 -> Position [m]/1
  Demux/2 -> Initial/2(DeltaPos)
  "DS3002POS_B1_C1 "/1 -> Demux/1
  ResetEnc/1 -> "DS3002SET_POS_B1_C1 "/Trigger
  ZP/1 -> AbsPosition/1
  Initial/1(Pos_offset) -> AbsPosition/3
  Init/1 -> Initial/3(Input)

== system LinMotAct_total/Actuator/Motor_B/Outputs to Amplifier ==
  Motor current [A] : Inport
  Current2V : Gain  Gain=10/3  SaturateOnIntegerOverflow=on  OutDataTypeStr=Inherit: Same as input  ParamDataTypeStr=Inherit: Same as input
  DS2102_B1 : rtilibm/DS2102/DS2102_B1  BoardNo=1  Range=[10 10 10 10 10 10]  IOErrorMode=[1 1 1 1 1 1]  DeglitcherMode=[0 0 0 0 0 0]  InitValue=[0 0 0 0 0 0]  TermMode=[1 1 1 1 1 1]  TermValue=[0 0 0 0 0 0]  DialogFcn=gui2102  UnitName={'DS2102_B'}  UnitValues={ 1 }  DSProperties=struct('RTI',struct('Version',uint32(1),'BlockType',struct('isSLSource',uint8(0),'isSLSink',uint8(1),'isHWSource',uint8(0),'isHWSink',uint8(1),'isSetup',uint8(0),'isInline',uint8(1),'isNonInline',uint8(0),'isInterrupt',uint8(0),'isChannelwise',uint8(0)),'IOBoardType','DS2102','UnitType','DAC','Identifier','DAC','DialogType','ML','BlockSet','NONE','SlaveProcessor','NONE'))
      settings: SourceProductName=dSPACE RTI1005
  DSPscale : Gain  Gain=1/10  SaturateOnIntegerOverflow=on  OutDataTypeStr=Inherit: Same as input  ParamDataTypeStr=Inherit: Same as input
  Saturation : Saturate  UpperLimit=3  LowerLimit=-3
  wires:
  Saturation/1 -> Current2V/1
  Current2V/1 -> DSPscale/1
  Motor current [A]/1 -> Saturation/1
  DSPscale/1 -> DS2102_B1/2

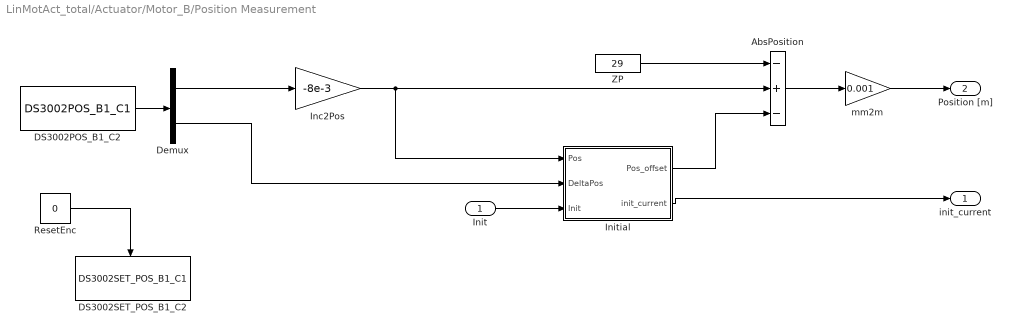
== system LinMotAct_total/Actuator/Motor_B/Position Measurement ==
  Init : Inport
  AbsPosition : Sum  Inputs=-+-  SaturateOnIntegerOverflow=on
  DS3002POS_B1_C2 : rti3002t2lib/DS3002POS_B1_C1  BoardNo=1  ChannelNo=2  LineSubdivNumOf=1  Reserved1=[]  Reserved2=[]  Reserved3=[]  Reserved4=[]  DialogFcn=gui3002pos_c_t2  UnitName={'DS3002POS_B', '_C'}  UnitValues="{ 1  2 }"  DSProperties=struct('RTI',struct('Version',uint32(1),'BlockType',struct('isSLSource',uint8(1),'isSLSink',uint8(0),'isHWSource',uint8(1),'isHWSink',uint8(0),'isSetup',uint8(0),'isInline',uint8(1),'isNonInline',uint8(0),'isInterrupt',uint8(0),'isChannelwise',uint8(1)),'IOBoardType','DS3002','UnitType','ENC','Identifier','ENCPOSCHT2','DialogType','ML','BlockSet','NONE','SlaveProcessor','NONE'))
  DS3002SET_POS_B1_C2 : rti3002t2lib/DS3002SET_POS_B1_C1  BoardNo=1  ChannelNo=2  PositionSetValue=0  Reserved1=[]  Reserved2=[]  Reserved3=[]  Reserved4=[]  DialogFcn=gui3002set_pos_c_t2  UnitName={'DS3002SET_POS_B', '_C'}  UnitValues="{ 1  2 }"  DSProperties=struct('RTI',struct('Version',uint32(1),'BlockType',struct('isSLSource',uint8(0),'isSLSink',uint8(1),'isHWSource',uint8(0),'isHWSink',uint8(0),'isSetup',uint8(0),'isInline',uint8(1),'isNonInline',uint8(0),'isInterrupt',uint8(0),'isChannelwise',uint8(1)),'IOBoardType','DS3002','UnitType','ENC','Identifier','ENCSETPOST2','DialogType','ML','BlockSet','NONE','SlaveProcessor','NONE'))
  Demux : Demux  Outputs=2
  Inc2Pos : Gain  Gain=-8e-3  SaturateOnIntegerOverflow=on  OutDataTypeStr=Inherit: Same as input  ParamDataTypeStr=Inherit: Same as input
  Initial : Subsystem
  ResetEnc : Constant  Value=0
  ZP : Constant  Value=29
  mm2m : Gain  Gain=0.001
  init_current : Outport  VectorParamsAs1DForOutWhenUnconnected=off
  Position [m] : Outport  Port=2  VectorParamsAs1DForOutWhenUnconnected=off
  wires:
  Demux/1 -> Inc2Pos/1
  AbsPosition/1 -> mm2m/1
  Inc2Pos/1 -> Initial/1(Pos), AbsPosition/2
  Initial/2(init_current) -> init_current/1
  mm2m/1 -> Position [m]/1
  Demux/2 -> Initial/2(DeltaPos)
  DS3002POS_B1_C2/1 -> Demux/1
  ResetEnc/1 -> DS3002SET_POS_B1_C2/Trigger
  ZP/1 -> AbsPosition/1
  Initial/1(Pos_offset) -> AbsPosition/3
  Init/1 -> Initial/3(Init)

== system LinMotAct_total/Actuator/Motor_C/Outputs to Amplifier ==
  Motor current [A] : Inport
  Current2V : Gain  Gain=10/3  SaturateOnIntegerOverflow=on  OutDataTypeStr=Inherit: Same as input  ParamDataTypeStr=Inherit: Same as input
  DS2102_B1 : rtilibm/DS2102/DS2102_B1  BoardNo=1  Range=[10 10 10 10 10 10]  IOErrorMode=[1 1 1 1 1 1]  DeglitcherMode=[0 0 0 0 0 0]  InitValue=[0 0 0 0 0 0]  TermMode=[1 1 1 1 1 1]  TermValue=[0 0 0 0 0 0]  DialogFcn=gui2102  UnitName={'DS2102_B'}  UnitValues={ 1 }  DSProperties=struct('RTI',struct('Version',uint32(1),'BlockType',struct('isSLSource',uint8(0),'isSLSink',uint8(1),'isHWSource',uint8(0),'isHWSink',uint8(1),'isSetup',uint8(0),'isInline',uint8(1),'isNonInline',uint8(0),'isInterrupt',uint8(0),'isChannelwise',uint8(0)),'IOBoardType','DS2102','UnitType','DAC','Identifier','DAC','DialogType','ML','BlockSet','NONE','SlaveProcessor','NONE'))
      settings: SourceProductName=dSPACE RTI1005
  DSPscale : Gain  Gain=1/10  SaturateOnIntegerOverflow=on  OutDataTypeStr=Inherit: Same as input  ParamDataTypeStr=Inherit: Same as input
  Saturation : Saturate  UpperLimit=3  LowerLimit=-3
  wires:
  Saturation/1 -> Current2V/1
  Current2V/1 -> DSPscale/1
  Motor current [A]/1 -> Saturation/1
  DSPscale/1 -> DS2102_B1/3

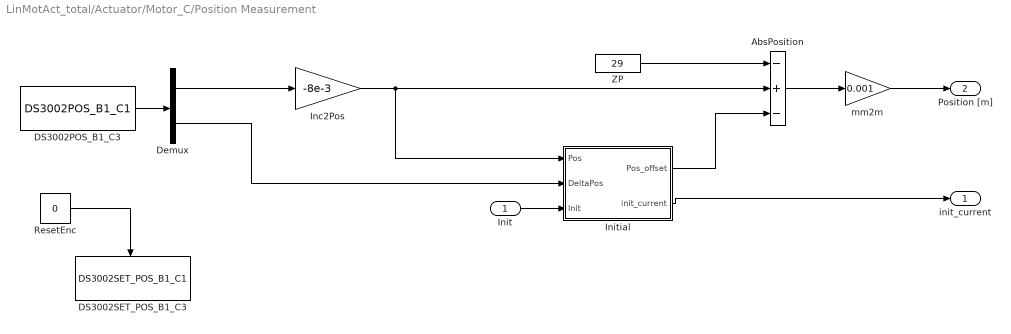
== system LinMotAct_total/Actuator/Motor_C/Position Measurement ==
  Init : Inport
  AbsPosition : Sum  Inputs=-+-  SaturateOnIntegerOverflow=on
  DS3002POS_B1_C3 : rti3002t2lib/DS3002POS_B1_C1  BoardNo=1  ChannelNo=3  LineSubdivNumOf=1  Reserved1=[]  Reserved2=[]  Reserved3=[]  Reserved4=[]  DialogFcn=gui3002pos_c_t2  UnitName={'DS3002POS_B', '_C'}  UnitValues="{ 1  3 }"  DSProperties=struct('RTI',struct('Version',uint32(1),'BlockType',struct('isSLSource',uint8(1),'isSLSink',uint8(0),'isHWSource',uint8(1),'isHWSink',uint8(0),'isSetup',uint8(0),'isInline',uint8(1),'isNonInline',uint8(0),'isInterrupt',uint8(0),'isChannelwise',uint8(1)),'IOBoardType','DS3002','UnitType','ENC','Identifier','ENCPOSCHT2','DialogType','ML','BlockSet','NONE','SlaveProcessor','NONE'))
  DS3002SET_POS_B1_C3 : rti3002t2lib/DS3002SET_POS_B1_C1  BoardNo=1  ChannelNo=3  PositionSetValue=0  Reserved1=[]  Reserved2=[]  Reserved3=[]  Reserved4=[]  DialogFcn=gui3002set_pos_c_t2  UnitName={'DS3002SET_POS_B', '_C'}  UnitValues="{ 1  3 }"  DSProperties=struct('RTI',struct('Version',uint32(1),'BlockType',struct('isSLSource',uint8(0),'isSLSink',uint8(1),'isHWSource',uint8(0),'isHWSink',uint8(0),'isSetup',uint8(0),'isInline',uint8(1),'isNonInline',uint8(0),'isInterrupt',uint8(0),'isChannelwise',uint8(1)),'IOBoardType','DS3002','UnitType','ENC','Identifier','ENCSETPOST2','DialogType','ML','BlockSet','NONE','SlaveProcessor','NONE'))
  Demux : Demux  Outputs=2
  Inc2Pos : Gain  Gain=-8e-3  SaturateOnIntegerOverflow=on  OutDataTypeStr=Inherit: Same as input  ParamDataTypeStr=Inherit: Same as input
  Initial : Subsystem
  ResetEnc : Constant  Value=0
  ZP : Constant  Value=29
  mm2m : Gain  Gain=0.001
  init_current : Outport  VectorParamsAs1DForOutWhenUnconnected=off
  Position [m] : Outport  Port=2  VectorParamsAs1DForOutWhenUnconnected=off
  wires:
  Demux/1 -> Inc2Pos/1
  AbsPosition/1 -> mm2m/1
  Inc2Pos/1 -> Initial/1(Pos), AbsPosition/2
  Initial/2(init_current) -> init_current/1
  mm2m/1 -> Position [m]/1
  Demux/2 -> Initial/2(DeltaPos)
  DS3002POS_B1_C3/1 -> Demux/1
  ResetEnc/1 -> DS3002SET_POS_B1_C3/Trigger
  ZP/1 -> AbsPosition/1
  Initial/1(Pos_offset) -> AbsPosition/3
  Init/1 -> Initial/3(Init)

== system LinMotAct_total/RTI Data/RTI Data Store/RTI Data Store ==
  RTI Data Store : Subsystem  mask(RTI_DATA_STORE){}
      mask help:
      | RTI Data Store Block. This block is used by RTI to store internal model dependent data. Deleting this block will result in data loss.
      |
      | NEVER DELETE, COPY, OR MODIFY THIS BLOCK!
      mask Help:
      | RTI Data Store Block. This block is used by RTI to store internal model dependent data. Deleting this block will result in data loss.
      | 
      | NEVER DELETE, COPY, OR MODIFY THIS BLOCK!
      mask Display: text(0.5, 0.5, ' ', 'HorizontalAlignment', 'center');

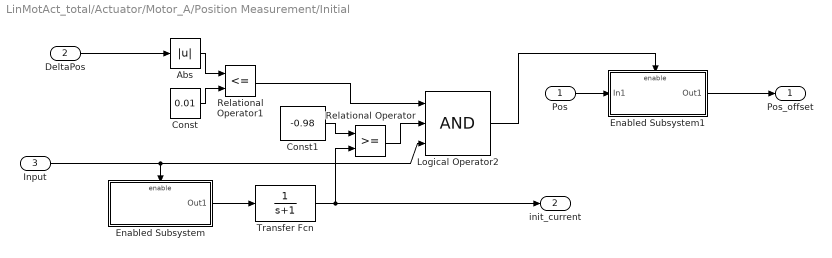
== system LinMotAct_total/Actuator/Motor_A/Position Measurement/Initial ==
  Pos : Inport
  DeltaPos : Inport  Port=2
  Input : Inport  Port=3
  Abs : Abs  SaturateOnIntegerOverflow=on
  Const : Constant  Value=0.01
  Const1 : Constant  Value=-0.98
  Enabled Subsystem : Subsystem  TreatAsAtomicUnit=on
  Enabled Subsystem1 : Subsystem  TreatAsAtomicUnit=on
  Logical Operator2 : Logic  Inputs=3  AllPortsSameDT=off
  Relational Operator : RelationalOperator  RndMeth=Nearest
  Relational Operator1 : RelationalOperator  Operator=<=  RndMeth=Nearest
  Transfer Fcn : TransferFcn  Denominator=[1 1]
  Pos_offset : Outport  VectorParamsAs1DForOutWhenUnconnected=off
  init_current : Outport  Port=2  VectorParamsAs1DForOutWhenUnconnected=off
  wires:
  Enabled Subsystem/1(Out1) -> Transfer Fcn/1
  Transfer Fcn/1 -> Relational Operator/2, init_current/1
  Input/1 -> Enabled Subsystem/Enable, Logical Operator2/3
  Const1/1 -> Relational Operator/1
  Abs/1 -> Relational Operator1/1
  Const/1 -> Relational Operator1/2
  Relational Operator1/1 -> Logical Operator2/1
  Relational Operator/1 -> Logical Operator2/2
  DeltaPos/1 -> Abs/1
  Logical Operator2/1 -> Enabled Subsystem1/Enable
  Pos/1 -> Enabled Subsystem1/1(In1)
  Enabled Subsystem1/1(Out1) -> Pos_offset/1

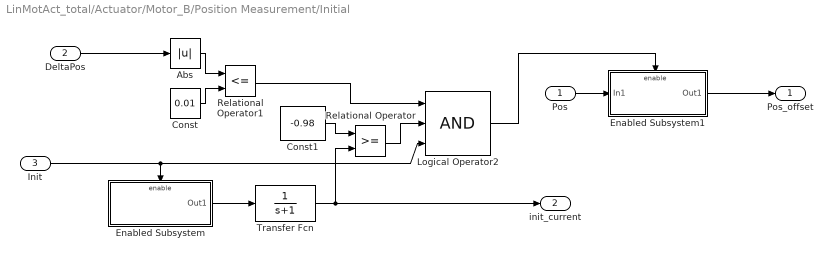
== system LinMotAct_total/Actuator/Motor_B/Position Measurement/Initial ==
  Pos : Inport
  DeltaPos : Inport  Port=2
  Init : Inport  Port=3
  Abs : Abs  SaturateOnIntegerOverflow=on
  Const : Constant  Value=0.01
  Const1 : Constant  Value=-0.98
  Enabled Subsystem : Subsystem  TreatAsAtomicUnit=on
  Enabled Subsystem1 : Subsystem  TreatAsAtomicUnit=on
  Logical Operator2 : Logic  Inputs=3  AllPortsSameDT=off
  Relational Operator : RelationalOperator  RndMeth=Nearest
  Relational Operator1 : RelationalOperator  Operator=<=  RndMeth=Nearest
  Transfer Fcn : TransferFcn  Denominator=[1 1]
  Pos_offset : Outport  VectorParamsAs1DForOutWhenUnconnected=off
  init_current : Outport  Port=2  VectorParamsAs1DForOutWhenUnconnected=off
  wires:
  Enabled Subsystem/1(Out1) -> Transfer Fcn/1
  Transfer Fcn/1 -> Relational Operator/2, init_current/1
  Init/1 -> Enabled Subsystem/Enable, Logical Operator2/3
  Const1/1 -> Relational Operator/1
  Abs/1 -> Relational Operator1/1
  Const/1 -> Relational Operator1/2
  Relational Operator1/1 -> Logical Operator2/1
  Relational Operator/1 -> Logical Operator2/2
  DeltaPos/1 -> Abs/1
  Logical Operator2/1 -> Enabled Subsystem1/Enable
  Pos/1 -> Enabled Subsystem1/1(In1)
  Enabled Subsystem1/1(Out1) -> Pos_offset/1

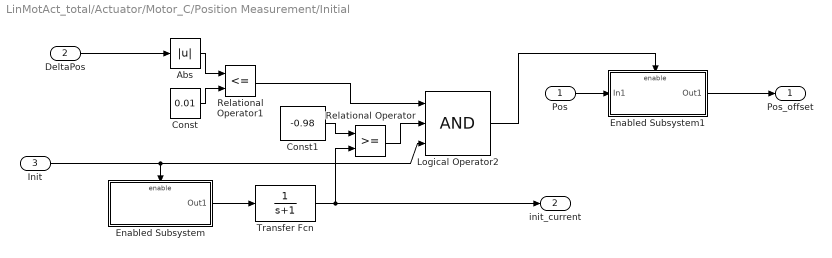
== system LinMotAct_total/Actuator/Motor_C/Position Measurement/Initial ==
  Pos : Inport
  DeltaPos : Inport  Port=2
  Init : Inport  Port=3
  Abs : Abs  SaturateOnIntegerOverflow=on
  Const : Constant  Value=0.01
  Const1 : Constant  Value=-0.98
  Enabled Subsystem : Subsystem  TreatAsAtomicUnit=on
  Enabled Subsystem1 : Subsystem  TreatAsAtomicUnit=on
  Logical Operator2 : Logic  Inputs=3  AllPortsSameDT=off
  Relational Operator : RelationalOperator  RndMeth=Nearest
  Relational Operator1 : RelationalOperator  Operator=<=  RndMeth=Nearest
  Transfer Fcn : TransferFcn  Denominator=[1 1]
  Pos_offset : Outport  VectorParamsAs1DForOutWhenUnconnected=off
  init_current : Outport  Port=2  VectorParamsAs1DForOutWhenUnconnected=off
  wires:
  Enabled Subsystem/1(Out1) -> Transfer Fcn/1
  Transfer Fcn/1 -> Relational Operator/2, init_current/1
  Init/1 -> Enabled Subsystem/Enable, Logical Operator2/3
  Const1/1 -> Relational Operator/1
  Abs/1 -> Relational Operator1/1
  Const/1 -> Relational Operator1/2
  Relational Operator1/1 -> Logical Operator2/1
  Relational Operator/1 -> Logical Operator2/2
  DeltaPos/1 -> Abs/1
  Logical Operator2/1 -> Enabled Subsystem1/Enable
  Pos/1 -> Enabled Subsystem1/1(In1)
  Enabled Subsystem1/1(Out1) -> Pos_offset/1

== system LinMotAct_total/RTI Data/RTI Data Store/RTI Data Store/RTI Data Store ==
  RTI Data Store : Subsystem  mask(RTI_DATA_STORE){}
      mask help:
      | RTI Data Store Block. This block is used by RTI to store internal model dependent data. Deleting this block will result in data loss.
      |
      | NEVER DELETE, COPY, OR MODIFY THIS BLOCK!
      mask Help:
      | RTI Data Store Block. This block is used by RTI to store internal model dependent data. Deleting this block will result in data loss.
      | 
      | NEVER DELETE, COPY, OR MODIFY THIS BLOCK!
      mask Display: text(0.5, 0.5, ' ', 'HorizontalAlignment', 'center');

== system LinMotAct_total/Actuator/Motor_A/Position Measurement/Initial/Enabled Subsystem ==
  Enable : EnablePort  PropagateVarSize=During execution
  Constant : Constant  Value=-1
  Out1 : Outport  OutputWhenDisabled=reset  InitialOutput=[0]  VectorParamsAs1DForOutWhenUnconnected=off
  wires:
  Constant/1 -> Out1/1

== system LinMotAct_total/Actuator/Motor_A/Position Measurement/Initial/Enabled Subsystem1 ==
  In1 : Inport
  Enable : EnablePort  PropagateVarSize=During execution
  Out1 : Outport  InitialOutput=[0]  VectorParamsAs1DForOutWhenUnconnected=off
  wires:
  In1/1 -> Out1/1

== system LinMotAct_total/Actuator/Motor_B/Position Measurement/Initial/Enabled Subsystem ==
  Enable : EnablePort  PropagateVarSize=During execution
  Constant : Constant  Value=-1
  Out1 : Outport  OutputWhenDisabled=reset  InitialOutput=[0]  VectorParamsAs1DForOutWhenUnconnected=off
  wires:
  Constant/1 -> Out1/1

== system LinMotAct_total/Actuator/Motor_B/Position Measurement/Initial/Enabled Subsystem1 ==
  In1 : Inport
  Enable : EnablePort  PropagateVarSize=During execution
  Out1 : Outport  InitialOutput=[0]  VectorParamsAs1DForOutWhenUnconnected=off
  wires:
  In1/1 -> Out1/1

== system LinMotAct_total/Actuator/Motor_C/Position Measurement/Initial/Enabled Subsystem ==
  Enable : EnablePort  PropagateVarSize=During execution
  Constant : Constant  Value=-1
  Out1 : Outport  OutputWhenDisabled=reset  InitialOutput=[0]  VectorParamsAs1DForOutWhenUnconnected=off
  wires:
  Constant/1 -> Out1/1

== system LinMotAct_total/Actuator/Motor_C/Position Measurement/Initial/Enabled Subsystem1 ==
  In1 : Inport
  Enable : EnablePort  PropagateVarSize=During execution
  Out1 : Outport  InitialOutput=[0]  VectorParamsAs1DForOutWhenUnconnected=off
  wires:
  In1/1 -> Out1/1

== system LinMotAct_total/RTI Data/RTI Data Store/RTI Data Store/RTI Data Store/RTI Data Store ==

== matlab function LinMotAct_total/Actuator/MATLAB Function2 ==
  data: Delta_P_A input; Alpha_angle output; Delta_P_B input; Delta_P_C input; L_in1 input; L_in2 input; L_in3 input; Beta_angle output; Psi_angle output; T_back output
function [Alpha_angle,Beta_angle,Psi_angle,T_back]      = myfunc(Delta_P_A,Delta_P_B,Delta_P_C,L_in1,L_in2,L_in3)



%% Specification of the base plate and plate

%Location of motors on the base plate 
r_base = 0.17;               %radii of the base plate (m)
B1     = [r_base; 0; 0]      %position of motor wrt base plate origin
B2     = [-0.5*r_base; (sqrt(3)/2)*r_base; 0]  %120degrees wrt the position of first motor and base plate origin
B3     = [-0.5*r_base; -(sqrt(3)/2)*r_base; 0] %240 degrees wrt first motor and base plate origin

%Location of joints on the plate 
r_plate = 0.17;               %radii of the plate (m)
P1     = [r_plate; 0; 0];      %position of motor wrt base plate origin
P2     = [-0.5*r_plate; (sqrt(3)/2)*r_plate; 0];  %120degrees wrt the position of first motor and base plate origin
P3     = [-0.5*r_plate; -(sqrt(3)/2)*r_plate; 0]; %240 degrees wrt first motor and base plate origin

% distance from base plate origin(OXYZ) to plate origin(oxyz)
T = [0; 0; 0.322]                     %30 cm height from (OXYZ) to (oxyz)

%actuator plate connections in base frame
% P1b= B1+(L_in1)-T;
% P2b= B2+(L_in2)-T;
% P3b= B3+(L_in3)-T;

P1b= B1+(L_in1*(Delta_P_A))-T;
P2b= B2+(L_in2*(Delta_P_B))-T;
P3b= B3+(L_in3*(Delta_P_C))-T;

%base frame unit vectors
UnitX=[1;0;0];
UnitY=[0;1;0];
UnitZ=[0;0;1];
UnitXp=P1b/sqrt(dot(P1b,P1b));
UnitZp=cross(UnitXp,P3b);
UnitZp=UnitZp/sqrt(dot(UnitZp,UnitZp)); %now length 1
UnitYp=cross(UnitXp,UnitZp);

%this is according to https://en.wikipedia.org/wiki/Euler_angles, Tait-Bryn
%angles

Beta_angle=asin(-UnitXp(3))
Psi_angle=asin(UnitXp(2)/sqrt(1-UnitXp(3)^2))
Alpha_angle=asin(UnitYp(3)/sqrt(1-UnitXp(3)^2))

%Calculating rotation matrix with above angles
RotZ1  = [cos(Psi_angle) -sin(Psi_angle) 0;
         sin(Psi_angle)  cos(Psi_angle) 0;
          0          0      1];
      
%    Y rotation with angle beta
RotY1  = [cos(Beta_angle)       0         sin(Beta_angle);
             0                           1             0    ;
         -sin(Beta_angle)      0        cos(Beta_angle)];
    
%    X rotation with angle alpha
RotX1  = [1            0                                 0    ;
         0        cos(Alpha_angle)      -sin(Alpha_angle);
         0        sin(Alpha_angle)       cos(Alpha_angle)];

% Calculating back the T matrix which was the height between the base plate
% and plate. They must be the same.
Rm_times_P = RotZ1*RotY1*RotX1
T_back = L_in1+B1-(Rm_times_P*P1)

end

== matlab function LinMotAct_total/MATLAB Function3 ==
  data: xreceive input; x output; yreceive input; y output
function [x,y]  = fcn(xreceive,yreceive)

%camera:    xrange = [85,318], yrange = [25,259]
%origin = 205,145

if (((xreceive<=205)&&(xreceive>=85))&&((yreceive>=145)&&(yreceive<=259)))      %1st quad
    x = (1/6.15)*(205-xreceive);  % x = 180 >> (217-180)/5.94 = 6.22 cm
    %x_pos = x * cos(alpha);
    y = (1/5.86)*(yreceive-145);  % y = 200 >> (200-117)/6.92 = 11.99 cm
    %y_pos = y * cos(alpha);
    if (xreceive<85)              % if it goes beyond the range from the right side(1st quad)
        x = int16(19.5);            % x becmes the maximum
    end
    if (yreceive>259)             % if it goes beyond the range from the right side(1st quad)
        y = int16(19.5);            % y becmes the maximum
    end   
elseif (((xreceive>205)&&(xreceive<=318))&&((yreceive>145)&&(yreceive<259)))  %2nd quad
    x = (-1/6.15)*(xreceive-205);  % x = 250 >> 250-217/(-5.94) = -5.55 cm
    %x_pos = x * cos(alpha);
    y = (1/5.86)*(yreceive-145);    % y = 200 >> (200-117)/6.92 = 11.99 cm
    %y_pos = y * cos(alpha)
    if (xreceive>318)
        x = int16(-19.5);
    end
    if (yreceive>259)
        y = int16(19.5);
    end

elseif (((xreceive>205)&&(xreceive<318))&&((yreceive<145)&&(yreceive>=25)))   %3rd quad
    x = (-1/6.15)*(xreceive-205);   % x = 250 >> 250-217/(-5.94) = -5.55 cm
    %x_pos = x * cos(alpha);
    y = (-1/5.86)*(145-yreceive);   % y = 100 >> 117-100/(-6.62) = -2.45 cm
    %y_pos = y * cos(alpha);
    if (xreceive>318)
        x = int16(-19.5);
    end
    if (yreceive<25)
        y = int16(-19.5);
    end

else                                                                         %4th quad
    x = (1/6.15)*(205-xreceive);  % x = 180 >> (217-180)/5.94 = 6.22 cm 
    %x_pos = x * cos(alpha);
    y = (-1/5.86)*(145-yreceive);  % y = 100 >> 117-100/(-6.62) = -2.45 cm
    %y_pos = y * cos(alpha);
    if (xreceive<85)
        x = int16(19.5);
    end
    if (yreceive<25)
        y = int16(-19.5);
    end    

end

== matlab function LinMotAct_total/Subsystem2/ForwardPosData ==
  data: TXenable output; TXData output; BytesIn input size=[4 1]; numRXBytes input size=1; BytesOut output; prevBytesOut input; HS_state output; prevHS_state input
function [TXenable,TXData, BytesOut, HS_state]  = fcn(BytesIn, numRXBytes, prevBytesOut, prevHS_state)

%TXData=cast(TXData,'uint8');

ACK=239; %0xef;
RXRD=223; %0xcf;
DR=255; %0xff;

TXenable=0;
TXData=0;

HS_state=prevHS_state;
BytesOut=prevBytesOut;

switch HS_state
    case 0 %wait for Data Ready signal from PI
        if BytesIn(1)== DR || BytesIn(2)== DR || BytesIn(3)== DR || BytesIn(4)== DR
            HS_state=1;
        else
            HS_state=0;
        end
    case 1 %make ACK high
        TXData=ACK;
        TXenable=1;
        HS_state=2;
    case 2 %make ACK low
        TXenable=0;
        HS_state=3;
    case 3 % forward 4 bytes of position data
        if  numRXBytes==4
            BytesOut=BytesIn;
            HS_state=4;
        else
            HS_state=3;
        end
    case 4 % reading done, notify PI
        TXData=RXRD;
        TXenable=1;
        HS_state=5;
    case 5
        TXenable=0;
        HS_state=0;
end
